simulink model "asserv_etat_lqr_sim_r2019b"  (R2019b)
settings: Solver=VariableStepAuto  StartTime=0.0  StopTime=inf  RelTol=1e-10
values from neighbouring files (symbols this model uses):
  g = 0.01    [asserv_etat_etendu_ini.m]    (also in identification_ini.m = 0.008703; identification_opt.m = x(4))
  Kt = 0.5    [asserv_etat_etendu_ini.m]    (also in identification_ini.m; identification_opt.m)
  Kv = 35.0    (= 35)    [asserv_etat_etendu_ini.m]    (also in identification_ini.m = 45.608692; identification_opt.m = x(1))
  L = [L(2) L(1) L(3)]    [asserv_etat_etendu_ini.m]    (also in asserv_etat_ini.m = [1 0]; asserv_etat_lqr_ini.m)
  tau_e = 0.003    [asserv_etat_etendu_ini.m]    (also in identification_ini.m = 0.002853; identification_opt.m = x(3))
  tau_m = 0.015    [asserv_etat_etendu_ini.m]    (also in identification_ini.m = 0.015641; identification_opt.m = x(2))
  Te = 0.002    [asserv_avance_phase_ini.m]    (also in asserv_etat_etendu_ini.m; identification_ini.m; identification_opt.m)
settings Model: EnablePacing=on  Creator=collette  LastModifiedBy=collette
settings DataIOCC: SaveOutput=off  SignalLogging=off  DSMLogging=off  SaveTime=off  ReturnWorkspaceOutputs=off
settings DebuggingCC: SFMachineParentedDataDiag=error

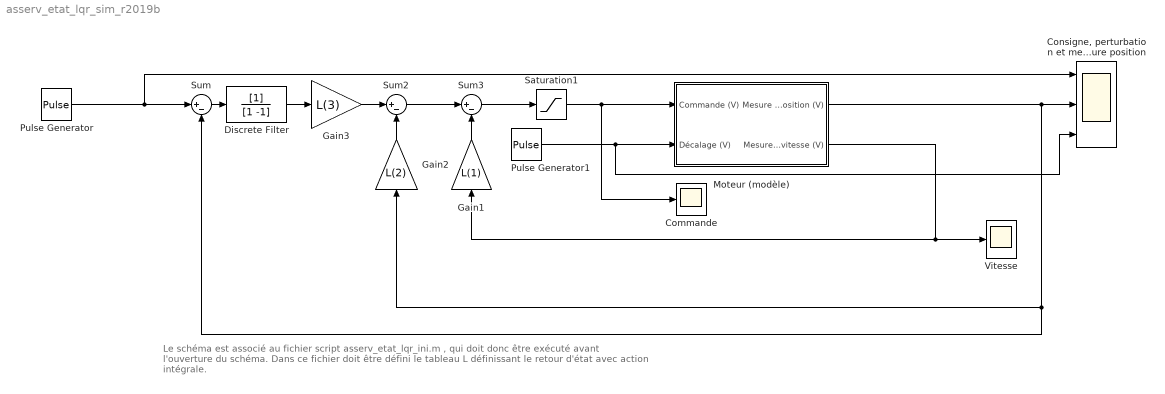
== system asserv_etat_lqr_sim_r2019b ==
  note: Le schéma est associé au fichier script asserv_etat_lqr_ini.m , qui doit donc être exécuté avant l'ouverture du schéma.
      | Dans ce fichier doit être défini le tableau L définissant le retour d'état avec action intégrale.
  Commande : Scope
  "Consigne, perturbation et mesure position" : Scope  NumInputPorts=3
  Discrete Filter : DiscreteFilter  Denominator=[1 -1]  SampleTime=Te
  Gain1 : Gain  Gain=L(1)
  Gain2 : Gain  Gain=L(2)
  Gain3 : Gain  Gain=L(3)
  Moteur (modèle) : Subsystem  mask{Parameter1=Kv, Parameter2=Kt, Parameter3=g, Parameter4=tau_m, Parameter5=tau_e, Parameter6=Te}
      mask prompts: Parameter1 "Kv"; Parameter2 "Kt"; Parameter3 "g"; Parameter4 "tau_m"; Parameter5 "tau_e"; Parameter6 "Te"
  Pulse Generator : DiscretePulseGenerator  PulseType=Time based  Amplitude=2  PulseWidth=50
  Pulse Generator1 : DiscretePulseGenerator  PulseType=Time based  Amplitude=4  PulseWidth=50  PhaseDelay=0.5
  Saturation1 : Saturate  UpperLimit=10  LowerLimit=-10
  Sum : Sum  Inputs=|+-
  Sum2 : Sum  Inputs=|+-
  Sum3 : Sum  Inputs=|+-
  Vitesse : Scope
  wires:
  Sum2/1 -> Sum3/1
  Gain1/1 -> Sum3/2
  Gain2/1 -> Sum2/2
  Gain3/1 -> Sum2/1
  Pulse Generator/1 -> Sum/1, "Consigne, perturbation et mesure position"/1
  Sum3/1 -> Saturation1/1
  Pulse Generator1/1 -> "Consigne, perturbation et mesure position"/3, Moteur (modèle)/2(Décalage (V))
  Sum/1 -> Discrete Filter/1
  Discrete Filter/1 -> Gain3/1
  Moteur (modèle)/1(Mesure position (V)) -> Gain2/1, Sum/2, "Consigne, perturbation et mesure position"/2
  Moteur (modèle)/2(Mesure vitesse (V)) -> Vitesse/1, Gain1/1
  Saturation1/1 -> Moteur (modèle)/1(Commande (V)), Commande/1

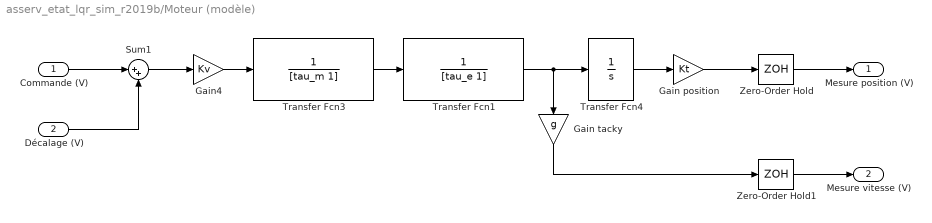
== system asserv_etat_lqr_sim_r2019b/Moteur (modèle) ==
  Commande (V) : Inport
  Décalage (V) : Inport  Port=2
  Gain position : Gain  Gain=Kt
  Gain tacky : Gain  Gain=g
  Gain4 : Gain  Gain=Kv
  Sum1 : Sum  Inputs=|++
  Transfer Fcn1 : TransferFcn  Denominator=[tau_e 1]
  Transfer Fcn3 : TransferFcn  Denominator=[tau_m 1]
  Transfer Fcn4 : TransferFcn  Denominator=[1 0]
  Zero-Order Hold : ZeroOrderHold  SampleTime=Te
  Zero-Order Hold1 : ZeroOrderHold  SampleTime=Te
  Mesure position (V) : Outport
  Mesure vitesse (V) : Outport  Port=2
  wires:
  Gain tacky/1 -> Zero-Order Hold1/1
  Transfer Fcn3/1 -> Transfer Fcn1/1
  Transfer Fcn4/1 -> Gain position/1
  Gain position/1 -> Zero-Order Hold/1
  Gain4/1 -> Transfer Fcn3/1
  Commande (V)/1 -> Sum1/1
  Sum1/1 -> Gain4/1
  Décalage (V)/1 -> Sum1/2
  Transfer Fcn1/1 -> Transfer Fcn4/1, Gain tacky/1
  Zero-Order Hold/1 -> Mesure position (V)/1
  Zero-Order Hold1/1 -> Mesure vitesse (V)/1
